simulink model "JMAP_Postfilt_SEModelv1d1"  (R2019a)
settings: Solver=FixedStepDiscrete  StartTime=0.0  StopTime=stopTime  RelTol=1e-3
InitFcn:
  | JMAP_INIT
StopFcn:
  | % Calls predefined matlab function for data analysis
  | JMAP_STOP
values from neighbouring files (symbols this model uses):
  aa = 0.98.*ones(FFT_size, 1)    [JMAP_INIT.m]    (also in JMAP_Postfilt_SE_OG.m = 0.98; JMAP_Postfilt_SE_v3.m = 0.98; JMAP_dataExport.m = 0.98; block_verScript.m = 0.98*ones(nSamp, FFT_size))
  beta = 2    [JMAP_INIT.m]    (also in JMAP_Postfilt_SE_OG.m; JMAP_dataExport.m; block_verScript.m = 2*ones(nSamp, FFT_size); ksi_verScript.m = 2*ones(nSamp, FFT_size))
  DPRAM1_size = FFT_size*2    (= 128)    [JMAP_INIT.m]
  FFT_frame_shift = FFT_size/4    (= 16)    [JMAP_INIT.m]
  FFT_size = 64    [FIR_filterTestm.m]    (also in JMAP_INIT.m; blockVerification.m; block_verScript.m; ksi_verScript.m)
  frameMag_initCond = abs(fft(sp(1:FFT_size), FFT_size))'    [JMAP_INIT.m]
  Fs = 48000    [FIR_filterTestm.m]    (also in JMAP_INIT.m; blockVerification.m; block_verScript.m; ksi_verScript.m)
  ksiInit = aa + (1-aa).*max(pSNR - 1, 0)    [JMAP_INIT.m]
  noiseVarianceInit = JMAP_noiseCalc(x)    [JMAP_INIT.m]
  SysRate_Upsample_Factor = 32    [JMAP_INIT.m]
  Ts = 1/Fs    (= 2.08333333333e-05)    [FIR_filterTestm.m]    (also in JMAP_INIT.m; blockVerification.m; block_verScript.m; ksi_verScript.m)
undefined symbols (not defined in the file or in its folder): Fs_in, magnitude
libraries: hdlsllib x16, simulink x7, dspxfrm3 x2, dspsigops x2
settings Model: Creator=Ross_admin  LastModifiedBy=Showi
settings DataIOCC: ReturnWorkspaceOutputs=off
settings OptimizationCC: BlockReduction=off  ConditionallyExecuteInputs=off  DefaultParameterBehavior=Inlined
settings DebuggingCC: AlgebraicLoopMsg=error  SingleTaskRateTransMsg=error  UnderSpecifiedDimensionMsg=warning  ArithmeticOperatorsInVariantConditions=warning
settings HardwareCC: ProdBitPerPointer=32  ProdBitPerSizeT=32  ProdBitPerPtrDiffT=32  ProdLargestAtomicFloat=None  ProdIntDivRoundTo=Undefined  ProdEndianess=Unspecified  ProdWordSize=32  ProdHWDeviceType=ASIC/FPGA->ASIC/FPGA  TargetBitPerPointer=64  TargetBitPerSizeT=64  TargetBitPerPtrDiffT=64  TargetLongLongMode=on  TargetIntDivRoundTo=Zero  TargetEndianess=LittleEndian  TargetWordSize=64  TargetHWDeviceType=Custom Processor->MATLAB Host Computer  ProdEqTarget=off
settings SFSimCC: SimUseLocalCustomCode=off
settings RTWCC: RTWUseLocalCustomCode=off
settings CodeAppCC: StateflowObjectComments=on

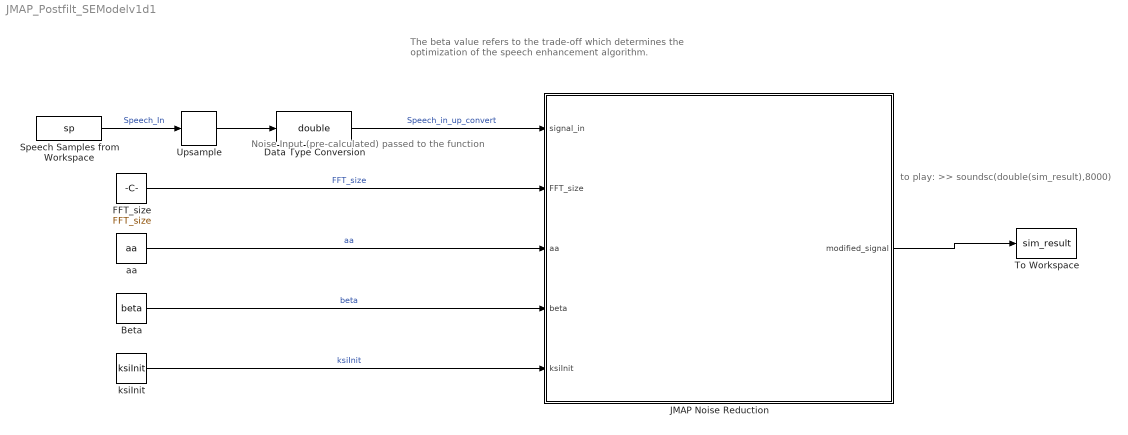
== system JMAP_Postfilt_SEModelv1d1 ==
  note: Noise Input (pre-calculated) passed to the function
  note: The beta value refers to the trade-off which determines the
      | optimization of the speech enhancement algorithm.
  note: to play: >> soundsc(double(sim_result),8000)
  Beta : Constant  Value=beta  SampleTime=Ts*2
  Data Type Conversion : DataTypeConversion  OutDataTypeStr=double
  FFT_size : Constant  Value=FFT_size  SampleTime=Ts*2
  JMAP Noise Reduction : Subsystem  TreatAsAtomicUnit=on
  Speech Samples from Workspace : FromWorkspace  VariableName=sp  SampleTime=Ts
  To Workspace : ToWorkspace  VariableName=sim_result  SampleTime=-1
  Upsample : dspsigops/Upsample  N=Fs/Fs_in  phase=0  RateOptions=Allow multirate processing  ic=0  mode=Unused parameter value
  aa : Constant  Value=aa  SampleTime=Ts*2
  ksiInit : Constant  Value=ksiInit  SampleTime=Ts*2
  wires:
  Speech Samples from Workspace/1 -> Upsample/1  "Speech_In"
  JMAP Noise Reduction/1(modified_signal) -> To Workspace/1
  Data Type Conversion/1 -> JMAP Noise Reduction/1(signal_in)  "Speech_in_up_convert"
  Upsample/1 -> Data Type Conversion/1
  Beta/1 -> JMAP Noise Reduction/4(beta)  "beta"
  aa/1 -> JMAP Noise Reduction/3(aa)  "aa"
  FFT_size/1 -> JMAP Noise Reduction/2(FFT_size)  "FFT_size"
  ksiInit/1 -> JMAP Noise Reduction/5(ksiInit)  "ksiInit"

== system JMAP_Postfilt_SEModelv1d1/JMAP Noise Reduction ==
  signal_in : Inport
  FFT_size : Inport  Port=2
  aa : Inport  Port=3
  beta : Inport  Port=4
  ksiInit : Inport  Port=5
  Analysis : Subsystem
  Frequency_Domain_Processing : Subsystem
  Synthesis : Subsystem
  modified_signal : Outport
  wires:
  signal_in/1 -> Analysis/1(Signal_in)
  Analysis/1(FFT_data) -> Frequency_Domain_Processing/5(FFT_results)
  Analysis/2(FFT_valid) -> Frequency_Domain_Processing/6(valid_in)
  Frequency_Domain_Processing/1(frequency_mods) -> Synthesis/1(FFT_data_mods)
  Frequency_Domain_Processing/2(valid_out) -> Synthesis/2(FFT_valid)
  Synthesis/1(modified_signal_out) -> modified_signal/1
  Analysis/3(FFT_frame_pulse) -> Synthesis/3(FFT_frame_pulse)  "FFT_framePulse"
  FFT_size/1 -> Frequency_Domain_Processing/1(FFT_size)
  aa/1 -> Frequency_Domain_Processing/2(aa)
  beta/1 -> Frequency_Domain_Processing/3(beta)
  ksiInit/1 -> Frequency_Domain_Processing/4(ksiInit)

== system JMAP_Postfilt_SEModelv1d1/JMAP Noise Reduction/Analysis ==
  note: Hanning window is applied
  Signal_in : Inport
  Data Type Conversion : DataTypeConversion  OutDataTypeStr=double
  FFT : dspxfrm3/FFT HDL Optimized  FFTLength=FFT_size  Architecture=Burst Radix 2  ComplexMultiplication=Use 4 multipliers and 2 adders  BitReversedOutput=off  BitReversedInput=off  Normalize=off  SimulateUsing=Code generation  RoundingMethod=Floor  ResetInputPort=off  StartOutputPort=off  EndOutputPort=off
      settings: SourceProductName=DSP System Toolbox  SourceProductBaseCode=DS
  FFT Frame Buffering : Subsystem
  Terminator6 : Terminator
  FFT_data : Outport
  FFT_valid : Outport  Port=2
  FFT_frame_pulse : Outport  Port=3
  wires:
  FFT/3 -> Terminator6/1
  FFT Frame Buffering/3(FFT_Frame_Start_Pulse) -> FFT_frame_pulse/1
  Signal_in/1 -> FFT Frame Buffering/1(Sample_Data_in)
  FFT Frame Buffering/2(Valid_to_FFT) -> FFT/2
  FFT Frame Buffering/1(Data_to_FFT) -> FFT/1
  Data Type Conversion/1 -> FFT_data/1
  FFT/2 -> FFT_valid/1
  FFT/1 -> Data Type Conversion/1

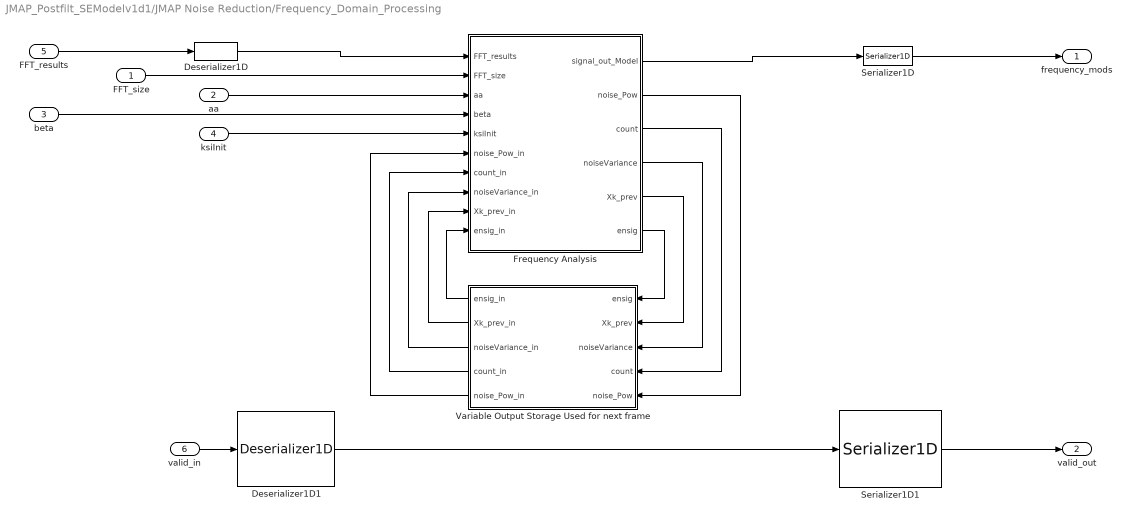
== system JMAP_Postfilt_SEModelv1d1/JMAP Noise Reduction/Frequency_Domain_Processing ==
  FFT_size : Inport
  aa : Inport  Port=2
  beta : Inport  Port=3
  ksiInit : Inport  Port=4
  FFT_results : Inport  Port=5
  valid_in : Inport  Port=6
  Deserializer1D : hdlsllib/HDL Operations/Deserializer1D  Ratio=FFT_size  IdleCycles=0  InitialCondition=0  startIn=off  validIn=off  validOut=off  inputDataDimensions=-1  inputSampleTime=-1  inputSignalType=auto
      settings: SourceProductName=HDL Coder  SourceProductBaseCode=HD
  Deserializer1D1 : hdlsllib/HDL Operations/Deserializer1D  Ratio=FFT_size  IdleCycles=0  InitialCondition=0  startIn=off  validIn=off  validOut=off  inputDataDimensions=-1  inputSampleTime=-1  inputSignalType=auto
      settings: SourceProductName=HDL Coder  SourceProductBaseCode=HD
  Frequency Analysis : Subsystem  TreatAsAtomicUnit=on
  Serializer1D : hdlsllib/HDL Operations/Serializer1D  Ratio=FFT_size  IdleCycles=0  validIn=off  startOut=off  validOut=off  inputDataDimensions=-1  inputSampleTime=-1  inputSignalType=auto
      settings: SourceProductName=HDL Coder  SourceProductBaseCode=HD
  Serializer1D1 : hdlsllib/HDL Operations/Serializer1D  Ratio=FFT_size  IdleCycles=0  validIn=off  startOut=off  validOut=off  inputDataDimensions=-1  inputSampleTime=-1  inputSignalType=auto
      settings: SourceProductName=HDL Coder  SourceProductBaseCode=HD
  Variable Output Storage Used for next frame : Subsystem
  frequency_mods : Outport
  valid_out : Outport  Port=2
  wires:
  Deserializer1D1/1 -> Serializer1D1/1
  FFT_results/1 -> Deserializer1D/1
  Serializer1D/1 -> frequency_mods/1
  valid_in/1 -> Deserializer1D1/1
  Serializer1D1/1 -> valid_out/1
  Deserializer1D/1 -> Frequency Analysis/1(FFT_results)
  Frequency Analysis/1(signal_out_Model) -> Serializer1D/1
  Frequency Analysis/6(ensig) -> Variable Output Storage Used for next frame/1(ensig)
  Frequency Analysis/5(Xk_prev) -> Variable Output Storage Used for next frame/2(Xk_prev)
  Frequency Analysis/4(noiseVariance) -> Variable Output Storage Used for next frame/3(noiseVariance)
  Frequency Analysis/3(count) -> Variable Output Storage Used for next frame/4(count)
  Variable Output Storage Used for next frame/1(ensig_in) -> Frequency Analysis/10(ensig_in)
  Variable Output Storage Used for next frame/2(Xk_prev_in) -> Frequency Analysis/9(Xk_prev_in)
  Variable Output Storage Used for next frame/3(noiseVariance_in) -> Frequency Analysis/8(noiseVariance_in)
  Variable Output Storage Used for next frame/4(count_in) -> Frequency Analysis/7(count_in)
  Frequency Analysis/2(noise_Pow) -> Variable Output Storage Used for next frame/5(noise_Pow)
  Variable Output Storage Used for next frame/5(noise_Pow_in) -> Frequency Analysis/6(noise_Pow_in)
  FFT_size/1 -> Frequency Analysis/2(FFT_size)
  beta/1 -> Frequency Analysis/4(beta)
  aa/1 -> Frequency Analysis/3(aa)
  ksiInit/1 -> Frequency Analysis/5(ksiInit)

== system JMAP_Postfilt_SEModelv1d1/JMAP Noise Reduction/Synthesis ==
  note: Making the assumption here
      | that the frequency domain processing
      | preserved the complex conjugate pairs.
  note: See Note 1
  note: Note 1:
      | Reshape is to avoid a simulink error.
      | Adding a FIFO to the iFFT block causes the
      | iFFT to change its output datatypes,
      | i.e. the data and valid signals
      | become a [1x1] matrix (Simulink Bug).
      | This work around was given by Mathworks
      | tech support (March 16, 2018).
      | Matlab 2017b
  note: See Note 1
  FFT_data_mods : Inport
  FFT_valid : Inport  Port=2
  FFT_frame_pulse : Inport  Port=3
  Data Type Conversion1 : DataTypeConversion  Commented=through  OutDataTypeStr=fixdt(1,Wbits,Fbits)
  Get_Real : ComplexToRealImag
  Overlap_and_Add : Subsystem
  Reshape : Reshape
  Reshape1 : Reshape
  Terminator8 : Terminator
  Terminator9 : Terminator
  iFFT : dspxfrm3/IFFT HDL Optimized  FFTLength=FFT_size  Architecture=Burst Radix 2  ComplexMultiplication=Use 4 multipliers and 2 adders  BitReversedOutput=off  BitReversedInput=off  Normalize=on  SimulateUsing=Code generation  RoundingMethod=Floor  ResetInputPort=off  StartOutputPort=off  EndOutputPort=off
      settings: SourceProductName=DSP System Toolbox  SourceProductBaseCode=DS
  modified_signal_out : Outport
  wires:
  iFFT/3 -> Terminator8/1
  Reshape1/1 -> Overlap_and_Add/2(iFFT_Valid)
  Reshape/1 -> Overlap_and_Add/1(IFFT_Data)
  iFFT/2 -> Reshape1/1
  Overlap_and_Add/1(signal_out) -> Data Type Conversion1/1
  FFT_data_mods/1 -> iFFT/1
  Data Type Conversion1/1 -> modified_signal_out/1  "modified_signal_outt"
  iFFT/1 -> Get_Real/1
  Get_Real/1 -> Reshape/1
  Get_Real/2 -> Terminator9/1
  FFT_valid/1 -> iFFT/2
  FFT_frame_pulse/1 -> Overlap_and_Add/3(FFT_Frame_Pulse)

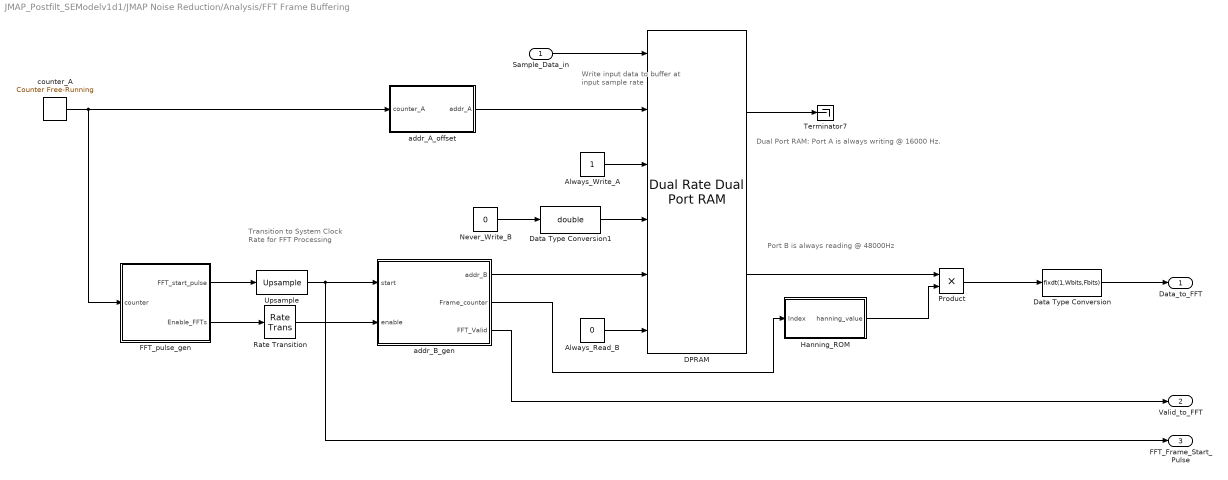
== system JMAP_Postfilt_SEModelv1d1/JMAP Noise Reduction/Analysis/FFT Frame Buffering ==
  note: Port B is always reading @ 48000Hz
  note: Dual Port RAM: Port A is always writing @ 16000 Hz.
  note: Transition to
      | System Clock Rate
      | for FFT Processing
  note: Write input data
      | to buffer at input
      | sample rate
  Sample_Data_in : Inport
  Always_Read_B : Constant  Value=0  OutDataTypeStr=boolean  SampleTime=Ts/SysRate_Upsample_Factor
  Always_Write_A : Constant  OutDataTypeStr=boolean  SampleTime=Ts
  DPRAM : hdlsllib/HDL RAMs/Dual Rate Dual Port RAM  ram_size=DPRAM1_address_size
      settings: SourceProductName=HDL Coder  SourceProductBaseCode=HD
  Data Type Conversion : DataTypeConversion  OutDataTypeStr=fixdt(1,Wbits,Fbits)
  Data Type Conversion1 : DataTypeConversion  OutDataTypeStr=double
  FFT_pulse_gen : Subsystem
  Hanning_ROM : Subsystem
  Never_Write_B : Constant  Value=0  OutDataTypeStr=fixdt(1,Wbits,Fbits)  SampleTime=Ts/SysRate_Upsample_Factor
  Product : Product
  Rate Transition : RateTransition  OutPortSampleTimeOpt=Multiple of input port sample time  OutPortSampleTimeMultiple=1/SysRate_Upsample_Factor
  Terminator7 : Terminator
  Upsample : dspsigops/Upsample  N=SysRate_Upsample_Factor  phase=0  RateOptions=Allow multirate processing  ic=0  mode=Unused parameter value
  addr_A_offset : Subsystem
  addr_B_gen : Subsystem
  counter_A : simulink/Sources/Counter Free-Running  NumBits=DPRAM1_address_size  tsamp=Ts
  Data_to_FFT : Outport
  Valid_to_FFT : Outport  Port=2
  FFT_Frame_Start_Pulse : Outport  Port=3
  wires:
  Always_Write_A/1 -> DPRAM/3
  Always_Read_B/1 -> DPRAM/6
  DPRAM/1 -> Terminator7/1
  addr_B_gen/3(FFT_Valid) -> Valid_to_FFT/1
  addr_B_gen/1(addr_B) -> DPRAM/5
  counter_A/1 -> addr_A_offset/1(counter_A), FFT_pulse_gen/1(counter)
  Sample_Data_in/1 -> DPRAM/1
  addr_A_offset/1(addr_A) -> DPRAM/2
  addr_B_gen/2(Frame_counter) -> Hanning_ROM/1(Index)
  Product/1 -> Data Type Conversion/1
  DPRAM/2 -> Product/1
  Hanning_ROM/1(hanning_value) -> Product/2
  Data Type Conversion/1 -> Data_to_FFT/1
  Rate Transition/1 -> addr_B_gen/2(enable)
  FFT_pulse_gen/1(FFT_start_pulse) -> Upsample/1
  FFT_pulse_gen/2(Enable_FFTs) -> Rate Transition/1
  Upsample/1 -> FFT_Frame_Start_Pulse/1, addr_B_gen/1(start)
  Data Type Conversion1/1 -> DPRAM/4
  Never_Write_B/1 -> Data Type Conversion1/1

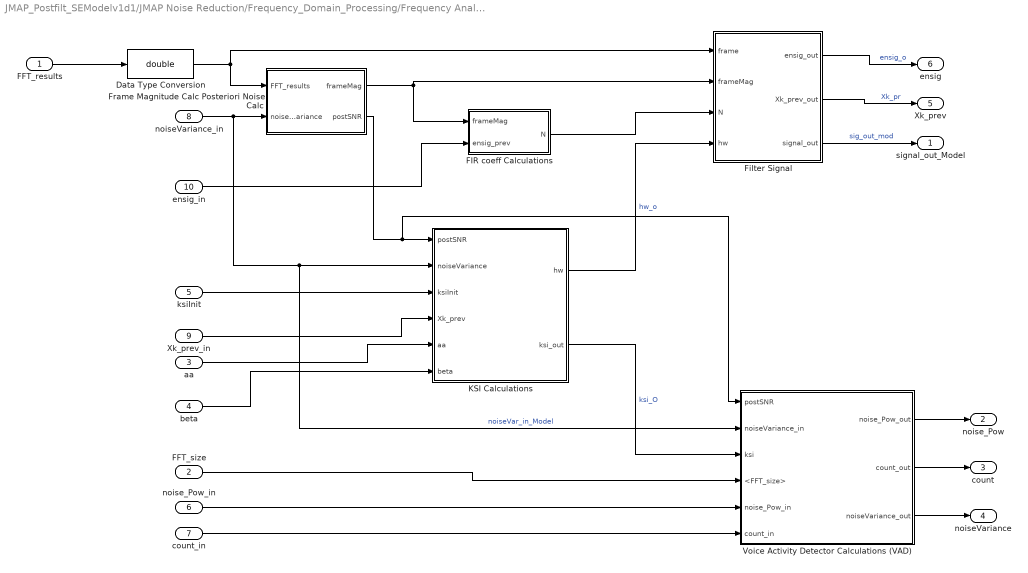
== system JMAP_Postfilt_SEModelv1d1/JMAP Noise Reduction/Frequency_Domain_Processing/Frequency Analysis ==
  FFT_results : Inport
  FFT_size : Inport  Port=2
  aa : Inport  Port=3
  beta : Inport  Port=4
  ksiInit : Inport  Port=5
  noise_Pow_in : Inport  Port=6
  count_in : Inport  Port=7
  noiseVariance_in : Inport  Port=8
  Xk_prev_in : Inport  Port=9
  ensig_in : Inport  Port=10
  Data Type Conversion : DataTypeConversion  OutDataTypeStr=double
  FIR coeff Calculations : Subsystem
  Filter Signal : Subsystem
  Frame Magnitude Calc Posteriori Noise Calc : Subsystem
  KSI Calculations : Subsystem
  Voice Activity Detector Calculations (VAD) : Subsystem
  signal_out_Model : Outport  InitialOutput=0
  noise_Pow : Outport  Port=2  InitialOutput=0
  count : Outport  Port=3  InitialOutput=0
  noiseVariance : Outport  Port=4  InitialOutput=0
  Xk_prev : Outport  Port=5  InitialOutput=0
  ensig : Outport  Port=6  InitialOutput=0
  wires:
  noise_Pow_in/1 -> Voice Activity Detector Calculations (VAD)/5("noise_Pow_in ")
  count_in/1 -> Voice Activity Detector Calculations (VAD)/6(count_in)
  Voice Activity Detector Calculations (VAD)/3(noiseVariance_out) -> noiseVariance/1
  Voice Activity Detector Calculations (VAD)/2(count_out) -> count/1
  Voice Activity Detector Calculations (VAD)/1(noise_Pow_out) -> noise_Pow/1
  Filter Signal/2(Xk_prev_out) -> Xk_prev/1  "Xk_pr"
  Filter Signal/1(ensig_out) -> ensig/1  "ensig_o"
  Filter Signal/3(signal_out) -> signal_out_Model/1  "sig_out_mod"
  Frame Magnitude Calc Posteriori Noise Calc/1(frameMag) -> FIR coeff Calculations/1(frameMag), Filter Signal/2(frameMag)
  FIR coeff Calculations/1(N) -> Filter Signal/3(N)
  Frame Magnitude Calc Posteriori Noise Calc/2(postSNR) -> Voice Activity Detector Calculations (VAD)/1(postSNR), KSI Calculations/1(postSNR)
  FFT_size/1 -> Voice Activity Detector Calculations (VAD)/4(<FFT_size>)
  Xk_prev_in/1 -> KSI Calculations/4(Xk_prev)
  aa/1 -> KSI Calculations/5(aa)
  beta/1 -> KSI Calculations/6(beta)
  KSI Calculations/1(hw) -> Filter Signal/4(hw)  "hw_o"
  KSI Calculations/2(ksi_out) -> Voice Activity Detector Calculations (VAD)/3(ksi)  "ksi_O"
  noiseVariance_in/1 -> KSI Calculations/2(noiseVariance), Voice Activity Detector Calculations (VAD)/2(noiseVariance_in), Frame Magnitude Calc Posteriori Noise Calc/2(noiseVariance)  "noiseVar_in_Model"
  FFT_results/1 -> Data Type Conversion/1
  Data Type Conversion/1 -> Filter Signal/1(frame), Frame Magnitude Calc Posteriori Noise Calc/1(FFT_results)
  ksiInit/1 -> KSI Calculations/3(ksiInit)
  ensig_in/1 -> FIR coeff Calculations/2(ensig_prev)

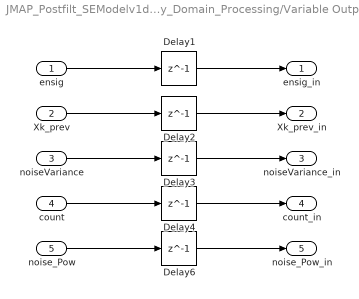
== system JMAP_Postfilt_SEModelv1d1/JMAP Noise Reduction/Frequency_Domain_Processing/Variable Output Storage Used for next frame ==
  ensig : Inport
  Xk_prev : Inport  Port=2
  noiseVariance : Inport  Port=3
  count : Inport  Port=4
  noise_Pow : Inport  Port=5
  Delay1 : Delay  DelayLength=1  InitialCondition=frameMag_initCond
  Delay2 : Delay  DelayLength=1  InitialCondition=zeros(FFT_size, 1)
  Delay3 : Delay  DelayLength=1  InitialCondition=noiseVarianceInit
  Delay4 : Delay  DelayLength=1  InitialCondition=1
  Delay6 : Delay  DelayLength=1  InitialCondition=zeros(FFT_size, 1)
  ensig_in : Outport
  Xk_prev_in : Outport  Port=2
  noiseVariance_in : Outport  Port=3
  count_in : Outport  Port=4
  noise_Pow_in : Outport  Port=5
  wires:
  ensig/1 -> Delay1/1
  Delay1/1 -> ensig_in/1
  Xk_prev/1 -> Delay2/1
  Delay2/1 -> Xk_prev_in/1
  noiseVariance/1 -> Delay3/1
  Delay3/1 -> noiseVariance_in/1
  count/1 -> Delay4/1
  Delay4/1 -> count_in/1
  noise_Pow/1 -> Delay6/1
  Delay6/1 -> noise_Pow_in/1

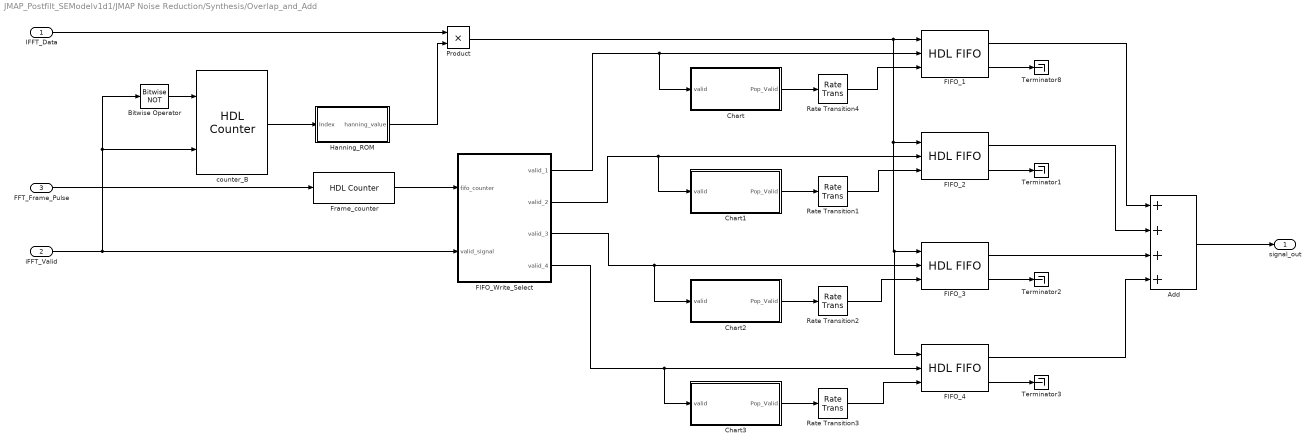
== system JMAP_Postfilt_SEModelv1d1/JMAP Noise Reduction/Synthesis/Overlap_and_Add ==
  IFFT_Data : Inport
  iFFT_Valid : Inport  Port=2
  FFT_Frame_Pulse : Inport  Port=3
  Add : Sum  Inputs=4
  Bitwise Operator : simulink/Logic and Bit Operations/Bitwise Operator  logicop=NOT  UseBitMask=off  BitMask=bin2dec('11011001')  BitMaskRealWorld=Stored Integer
  Chart : Stateflow chart  TreatAsAtomicUnit=on
  Chart1 : Stateflow chart  TreatAsAtomicUnit=on
  Chart2 : Stateflow chart  TreatAsAtomicUnit=on
  Chart3 : Stateflow chart  TreatAsAtomicUnit=on
  FIFO_{1..4} (4 alike) : hdlsllib/HDL RAMs/HDL FIFO  fifo_size=FFT_size  ratio=SysRate_Upsample_Factor  push_msg=Warning  pop_msg=Warning  show_empty=off  show_full=on  show_num=off
      settings: SourceProductName=HDL Coder  SourceProductBaseCode=HD
  FIFO_Write_Select : MATLAB Function  TreatAsAtomicUnit=on
  Frame_counter : hdlsllib/Sources/HDL Counter  CountType=Free running  CountInit=2  CountStep=1  CountMax=1024  CountFromType=Initial value  CountFrom=2  CountResetPort=off  CountLoadPort=off  CountEnbPort=on  CountDirPort=off  CountDataType=Unsigned  CountWordLen=2  CountFracLen=0  CountSampTime=1
      settings: SourceProductBaseCode=HD
  Hanning_ROM : Subsystem
  Product : Product
  Rate Transition{1..4} (4 alike) : RateTransition  OutPortSampleTimeOpt=Multiple of input port sample time  OutPortSampleTimeMultiple=SysRate_Upsample_Factor
  Terminator{1..3,8} (4 alike) : Terminator
  counter_B : hdlsllib/Sources/HDL Counter  CountType=Count limited  CountInit=0  CountStep=1  CountMax=FFT_size  CountFromType=Initial value  CountFrom=0  CountResetPort=on  CountLoadPort=off  CountEnbPort=on  CountDirPort=off  CountDataType=Unsigned  CountWordLen=DPRAM1_address_size  CountFracLen=0  CountSampTime=1
      settings: SourceProductBaseCode=HD
  signal_out : Outport
  wires:
  FIFO_1/1 -> Add/1
  FIFO_3/1 -> Add/3
  FFT_Frame_Pulse/1 -> Frame_counter/1
  FIFO_2/1 -> Add/2
  FIFO_Write_Select/3(valid_3) -> Chart2/1(valid), FIFO_3/2
  FIFO_Write_Select/4(valid_4) -> Chart3/1(valid), FIFO_4/2
  FIFO_4/1 -> Add/4
  FIFO_Write_Select/1(valid_1) -> FIFO_1/2, Chart/1(valid)
  FIFO_Write_Select/2(valid_2) -> FIFO_2/2, Chart1/1(valid)
  Add/1 -> signal_out/1
  Frame_counter/1 -> FIFO_Write_Select/1(fifo_counter)
  FIFO_4/2 -> Terminator3/1
  FIFO_2/2 -> Terminator1/1
  FIFO_3/2 -> Terminator2/1
  Bitwise Operator/1 -> counter_B/1
  iFFT_Valid/1 -> counter_B/2, Bitwise Operator/1, FIFO_Write_Select/2(valid_signal)
  IFFT_Data/1 -> Product/1
  Product/1 -> FIFO_4/1, FIFO_3/1, FIFO_2/1, FIFO_1/1
  Hanning_ROM/1(hanning_value) -> Product/2
  counter_B/1 -> Hanning_ROM/1(Index)
  Chart/1(Pop_Valid) -> Rate Transition4/1
  Rate Transition4/1 -> FIFO_1/3
  FIFO_1/2 -> Terminator8/1
  Chart1/1(Pop_Valid) -> Rate Transition1/1
  Rate Transition1/1 -> FIFO_2/3
  Chart2/1(Pop_Valid) -> Rate Transition2/1
  Rate Transition2/1 -> FIFO_3/3
  Chart3/1(Pop_Valid) -> Rate Transition3/1
  Rate Transition3/1 -> FIFO_4/3

== system JMAP_Postfilt_SEModelv1d1/JMAP Noise Reduction/Analysis/FFT Frame Buffering/FFT_pulse_gen ==
  note: Don't send out start pulses until
      | circular buffer has filled.
  counter : Inport
  FFT_Frame_Pulse_Gen : Subsystem
  Subsystem : Subsystem
  FFT_start_pulse : Outport
  Enable_FFTs : Outport  Port=2
  wires:
  counter/1 -> FFT_Frame_Pulse_Gen/1("counter_value ")
  Subsystem/1(FFT_Frame_Start) -> FFT_start_pulse/1
  Subsystem/2(Enable_FFT_Frames) -> Enable_FFTs/1
  FFT_Frame_Pulse_Gen/1(Frame_Pulse) -> Subsystem/1(Frame_Pulse)

== system JMAP_Postfilt_SEModelv1d1/JMAP Noise Reduction/Analysis/FFT Frame Buffering/Hanning_ROM ==
  Index : Inport
  Lookup Table : Lookup_n-D  NumberOfTableDimensions=1  BreakpointsForDimension1=[0:FFT_size]  IndexSearchMethod=Evenly spaced points  Table=hanning(FFT_size+1)  InterpMethod=Flat  ExtrapMethod=Clip  DiagnosticForOutOfRangeInput=Error  UseLastTableValue=on  OutDataTypeStr=double  RndMeth=Simplest  InputSameDT=on
  Unit Delay : UnitDelay  SampleTime=-1  HasFrameUpgradeWarning=on
  hanning_value : Outport
  wires:
  Unit Delay/1 -> hanning_value/1
  Index/1 -> Lookup Table/1
  Lookup Table/1 -> Unit Delay/1

== system JMAP_Postfilt_SEModelv1d1/JMAP Noise Reduction/Analysis/FFT Frame Buffering/addr_A_offset ==
  note: Add 1 to counter since the read pointer (addr_B)
      | can catch the write pointer (addr_A) if
      | SysRate_Upsample_Factor is large enough
  counter_A : Inport
  Add : Sum  OutDataTypeStr=fixdt(0,DPRAM1_address_size,0)
  write_offset : Constant  OutDataTypeStr=fixdt(0,DPRAM1_address_size,0)  SampleTime=Ts
  addr_A : Outport
  wires:
  write_offset/1 -> Add/2
  Add/1 -> addr_A/1
  counter_A/1 -> Add/1

== system JMAP_Postfilt_SEModelv1d1/JMAP Noise Reduction/Analysis/FFT Frame Buffering/addr_B_gen ==
  start : Inport
  enable : Inport  Port=2
  Logical Operator1 : Logic  AllPortsSameDT=off  OutDataTypeStr=boolean
  addr_B_gen_enable : Subsystem
  counter_B : hdlsllib/Sources/HDL Counter  CountType=Free running  CountInit=DPRAM1_size-10  CountStep=1  CountMax=1024  CountFromType=Initial value  CountFrom=DPRAM1_size-10  CountResetPort=off  CountLoadPort=on  CountEnbPort=on  CountDirPort=off  CountDataType=Unsigned  CountWordLen=DPRAM1_address_size  CountFracLen=0  CountSampTime=1
      settings: SourceProductBaseCode=HD
  addr_B : Outport
  Frame_counter : Outport  Port=2
  FFT_Valid : Outport  Port=3
  wires:
  counter_B/1 -> addr_B/1
  start/1 -> counter_B/1, addr_B_gen_enable/1(start)
  addr_B_gen_enable/1(enable_B) -> Logical Operator1/1
  addr_B_gen_enable/2(Start_Address) -> counter_B/2
  enable/1 -> Logical Operator1/2
  addr_B_gen_enable/3(Frame_Index) -> Frame_counter/1
  Logical Operator1/1 -> FFT_Valid/1, counter_B/3

== system JMAP_Postfilt_SEModelv1d1/JMAP Noise Reduction/Frequency_Domain_Processing/Frequency Analysis/FIR coeff Calculations ==
  frameMag : Inport
  ensig_prev : Inport  Port=2
  Calculate Coeffs and Filter Length : Subsystem
  PR Calculations : Subsystem
  PRT Calculation : Subsystem
  N : Outport
  wires:
  ensig_prev/1 -> PR Calculations/1(ensig_prev)
  PR Calculations/1(PR) -> PRT Calculation/1(PR)
  Calculate Coeffs and Filter Length/1(N) -> N/1
  PRT Calculation/1(PRT) -> Calculate Coeffs and Filter Length/1(PRT)
  frameMag/1 -> PR Calculations/2(frameMag)

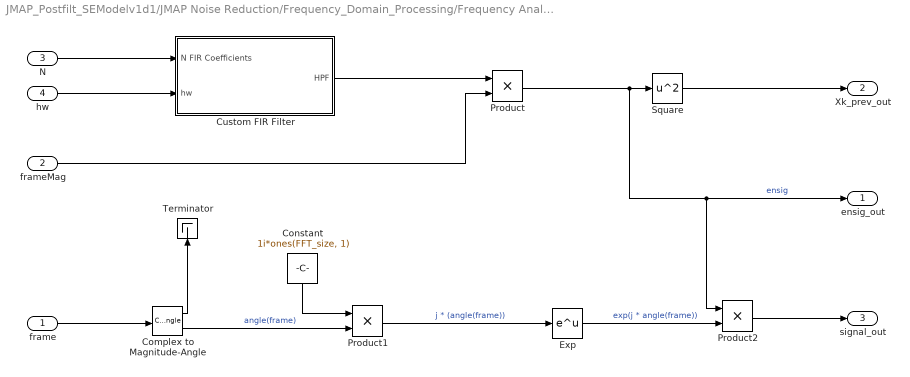
== system JMAP_Postfilt_SEModelv1d1/JMAP Noise Reduction/Frequency_Domain_Processing/Frequency Analysis/Filter Signal ==
  frame : Inport
  frameMag : Inport  Port=2
  N : Inport  Port=3
  hw : Inport  Port=4
  Complex to Magnitude-Angle : ComplexToMagnitudeAngle
  Constant : Constant  Value=1i*ones(FFT_size, 1)  SampleTime=-1
  Custom FIR Filter : Subsystem
  Exp : Math  SaturateOnIntegerOverflow=on
  Product : Product
  Product1 : Product
  Product2 : Product
  Square : Math  Operator=square  RndMeth=Zero  SaturateOnIntegerOverflow=on
  Terminator : Terminator
  ensig_out : Outport
  Xk_prev_out : Outport  Port=2
  signal_out : Outport  Port=3
  wires:
  Square/1 -> Xk_prev_out/1
  frameMag/1 -> Product/2
  Product1/1 -> Exp/1  "j * (angle(frame))"
  Constant/1 -> Product1/1
  Exp/1 -> Product2/2  "exp(j * angle(frame))"
  Product2/1 -> signal_out/1
  Complex to Magnitude-Angle/2 -> Product1/2  "angle(frame)"
  Complex to Magnitude-Angle/1 -> Terminator/1
  N/1 -> Custom FIR Filter/1(N FIR Coefficients)
  hw/1 -> Custom FIR Filter/2(hw)
  frame/1 -> Complex to Magnitude-Angle/1
  Product/1 -> Product2/1, ensig_out/1, Square/1  "ensig"
  Custom FIR Filter/1(HPF) -> Product/1

== system JMAP_Postfilt_SEModelv1d1/JMAP Noise Reduction/Frequency_Domain_Processing/Frequency Analysis/Frame Magnitude Calc Posteriori Noise Calc ==
  FFT_results : Inport
  noiseVariance : Inport  Port=2
  Subsystem1 : Subsystem
  Subsystem3 : Subsystem
  frameMag : Outport
  postSNR : Outport  Port=2
  wires:
  Subsystem3/2(frameMag) -> frameMag/1
  Subsystem3/1(framePower) -> Subsystem1/1(framePower)
  FFT_results/1 -> Subsystem3/1(FFT_results)
  noiseVariance/1 -> Subsystem1/2(noiseVariance)
  Subsystem1/1(postSNR) -> postSNR/1  "postSNR"

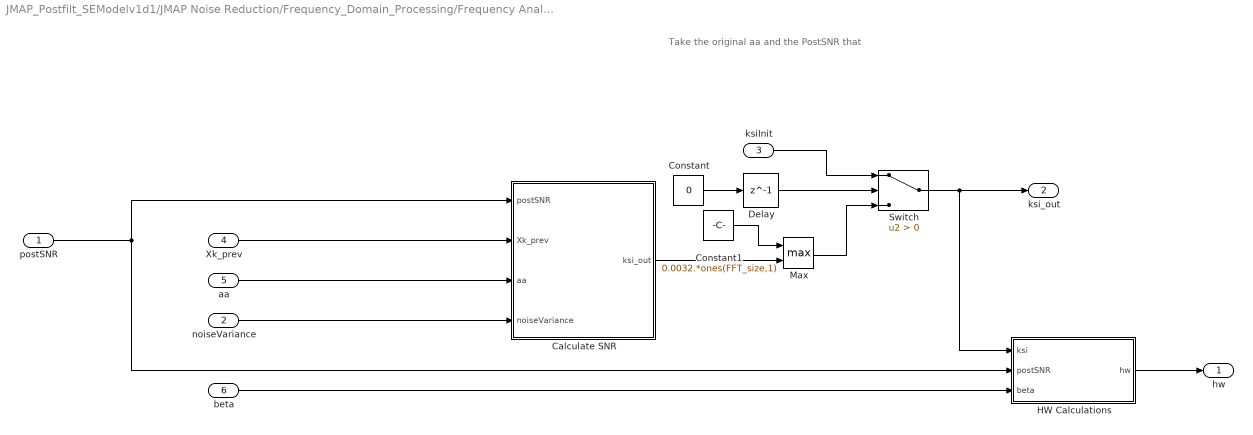
== system JMAP_Postfilt_SEModelv1d1/JMAP Noise Reduction/Frequency_Domain_Processing/Frequency Analysis/KSI Calculations ==
  note: Take the original aa and the PostSNR that
  postSNR : Inport
  noiseVariance : Inport  Port=2
  ksiInit : Inport  Port=3
  Xk_prev : Inport  Port=4
  aa : Inport  Port=5
  beta : Inport  Port=6
  Calculate SNR : Subsystem
  Constant : Constant  Value=0  SampleTime=-1
  Constant1 : Constant  Value=0.0032.*ones(FFT_size,1)  SampleTime=-1
  Delay : Delay  DelayLength=1  InitialCondition=1
  HW Calculations : Subsystem
  Max : MinMax  Function=max  Inputs=2
  Switch : Switch  Criteria=u2 > Threshold
  hw : Outport
  ksi_out : Outport  Port=2
  wires:
  noiseVariance/1 -> Calculate SNR/4(noiseVariance)
  beta/1 -> HW Calculations/3(beta)
  postSNR/1 -> HW Calculations/2(postSNR), Calculate SNR/1(postSNR)
  Xk_prev/1 -> Calculate SNR/2(Xk_prev)
  aa/1 -> Calculate SNR/3(aa)
  HW Calculations/1(hw) -> hw/1
  Switch/1 -> HW Calculations/1(ksi), ksi_out/1
  ksiInit/1 -> Switch/1
  Delay/1 -> Switch/2
  Constant/1 -> Delay/1
  Calculate SNR/1(ksi_out) -> Max/2
  Constant1/1 -> Max/1
  Max/1 -> Switch/3

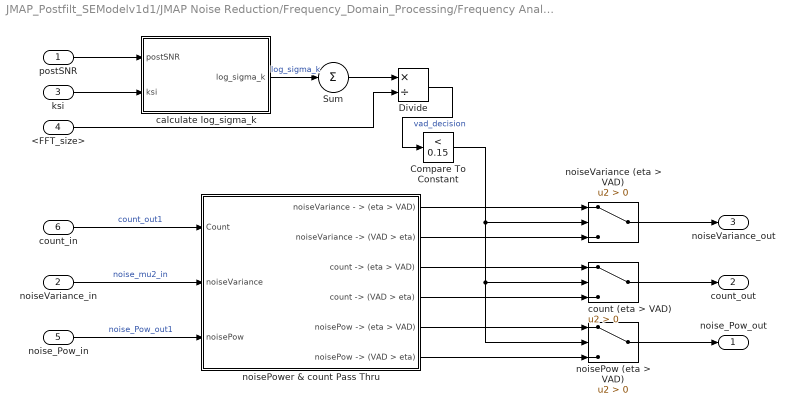
== system JMAP_Postfilt_SEModelv1d1/JMAP Noise Reduction/Frequency_Domain_Processing/Frequency Analysis/Voice Activity Detector Calculations (VAD) ==
  postSNR : Inport
  noiseVariance_in : Inport  Port=2
  ksi : Inport  Port=3
  <FFT_size> : Inport  Port=4
  "noise_Pow_in " : Inport  Port=5
  count_in : Inport  Port=6
  Compare To Constant : simulink/Logic and Bit Operations/Compare To Constant  relop=<  const=0.15  OutDataTypeStr=boolean
  Divide : Product  Inputs=*/  SaturateOnIntegerOverflow=on  RndMeth=Zero
  Sum : Sum  Inputs=+
  calculate log_sigma_k : Subsystem
  count (eta > VAD) : Switch  Criteria=u2 > Threshold
  noisePow (eta > VAD) : Switch  Criteria=u2 > Threshold
  noisePower & count Pass Thru : Subsystem
  noiseVariance (eta > VAD) : Switch  Criteria=u2 > Threshold
  noise_Pow_out : Outport  InitialOutput=0
  count_out : Outport  Port=2
  noiseVariance_out : Outport  Port=3
  wires:
  postSNR/1 -> calculate log_sigma_k/1(postSNR)
  ksi/1 -> calculate log_sigma_k/2(ksi)
  calculate log_sigma_k/1(log_sigma_k) -> Sum/1  "log_sigma_k"
  Sum/1 -> Divide/1
  <FFT_size>/1 -> Divide/2
  Divide/1 -> Compare To Constant/1  "vad_decision"
  noiseVariance_in/1 -> noisePower & count Pass Thru/2(noiseVariance)  "noise_mu2_in"
  "noise_Pow_in "/1 -> noisePower & count Pass Thru/3(noisePow)  "noise_Pow_out1"
  count_in/1 -> noisePower & count Pass Thru/1(Count)  "count_out1"
  Compare To Constant/1 -> noisePow (eta > VAD)/2, count (eta > VAD)/2, noiseVariance (eta > VAD)/2
  noisePower & count Pass Thru/1(noiseVariance - > (eta > VAD)) -> noiseVariance (eta > VAD)/1
  noisePower & count Pass Thru/2("noiseVariance -> (VAD > eta)") -> noiseVariance (eta > VAD)/3
  noisePower & count Pass Thru/3("count -> (eta > VAD)") -> count (eta > VAD)/1
  noisePower & count Pass Thru/4("count -> (VAD > eta)") -> count (eta > VAD)/3
  noiseVariance (eta > VAD)/1 -> noiseVariance_out/1
  count (eta > VAD)/1 -> count_out/1
  noisePow (eta > VAD)/1 -> noise_Pow_out/1
  noisePower & count Pass Thru/5("noisePow -> (eta > VAD)") -> noisePow (eta > VAD)/1
  noisePower & count Pass Thru/6("noisePow -> (VAD > eta)") -> noisePow (eta > VAD)/3

== system JMAP_Postfilt_SEModelv1d1/JMAP Noise Reduction/Synthesis/Overlap_and_Add/Hanning_ROM ==
  Index : Inport
  Lookup Table : Lookup_n-D  NumberOfTableDimensions=1  BreakpointsForDimension1=[0:FFT_size]  IndexSearchMethod=Evenly spaced points  Table=hanning(FFT_size+1)  InterpMethod=Flat  ExtrapMethod=Clip  DiagnosticForOutOfRangeInput=Error  UseLastTableValue=on  OutDataTypeStr=double  RndMeth=Simplest  InputSameDT=on
  Unit Delay : UnitDelay  SampleTime=-1  HasFrameUpgradeWarning=on
  hanning_value : Outport
  wires:
  Unit Delay/1 -> hanning_value/1
  Index/1 -> Lookup Table/1
  Lookup Table/1 -> Unit Delay/1

== system JMAP_Postfilt_SEModelv1d1/JMAP Noise Reduction/Analysis/FFT Frame Buffering/FFT_pulse_gen/FFT_Frame_Pulse_Gen ==
  "counter_value " : Inport
  Bit Slice : hdlsllib/Logic and Bit Operations/Bit Slice  lidx=log2(FFT_frame_shift)-1  ridx=0
  Compare To Zero : simulink/Logic and Bit Operations/Compare To Zero  relop===  OutDataTypeStr=boolean
  Frame_Pulse : Outport
  wires:
  "counter_value "/1 -> Bit Slice/1
  Compare To Zero/1 -> Frame_Pulse/1
  Bit Slice/1 -> Compare To Zero/1

== system JMAP_Postfilt_SEModelv1d1/JMAP Noise Reduction/Analysis/FFT Frame Buffering/FFT_pulse_gen/Subsystem ==
  note: Number of Frames
      | to wait before starting
  note: Start performing FFTs after enough data has filled the circular buffer.
      | This is due to the fact that we don't want the read pointer (addr_B)
      | to catch up with the  write pointer (addr_A) because if it does,
      | the DPRAM will throw an assertion error.
  Frame_Pulse : Inport
  Bitwise Operator : simulink/Logic and Bit Operations/Bitwise Operator  logicop=NOT  UseBitMask=off  BitMask=bin2dec('11011001')  BitMaskRealWorld=Stored Integer
  Compare To Constant : simulink/Logic and Bit Operations/Compare To Constant  relop=<  const=4  OutDataTypeStr=boolean
  Initial_frame_count : hdlsllib/Sources/HDL Counter  CountType=Count limited  CountInit=0  CountStep=1  CountMax=4  CountFromType=Specify  CountFrom=0  CountResetPort=off  CountLoadPort=off  CountEnbPort=on  CountDirPort=off  CountDataType=Unsigned  CountWordLen=5  CountFracLen=0  CountSampTime=1
      settings: SourceProductBaseCode=HD
  Logical Operator : Logic  AllPortsSameDT=off  OutDataTypeStr=boolean
  Logical Operator1 : Logic  AllPortsSameDT=off  OutDataTypeStr=boolean
  FFT_Frame_Start : Outport
  Enable_FFT_Frames : Outport  Port=2
  wires:
  Logical Operator1/1 -> FFT_Frame_Start/1
  Frame_Pulse/1 -> Logical Operator/2, Logical Operator1/1
  Initial_frame_count/1 -> Compare To Constant/1
  Logical Operator/1 -> Initial_frame_count/1
  Compare To Constant/1 -> Bitwise Operator/1, Logical Operator/1
  Bitwise Operator/1 -> Enable_FFT_Frames/1, Logical Operator1/2

== system JMAP_Postfilt_SEModelv1d1/JMAP Noise Reduction/Analysis/FFT Frame Buffering/addr_B_gen/addr_B_gen_enable ==
  start : Inport
  B_Enable_Counter : hdlsllib/Sources/HDL Counter  CountType=Count limited  CountInit=0  CountStep=1  CountMax=FFT_size  CountFromType=Specify  CountFrom=0  CountResetPort=on  CountLoadPort=off  CountEnbPort=on  CountDirPort=off  CountDataType=Unsigned  CountWordLen=DPRAM1_address_size  CountFracLen=0  CountSampTime=1
      settings: SourceProductBaseCode=HD
  Constant5 : Constant  Value=FFT_size  OutDataTypeStr=fixdt(0,11,0)  SampleTime=Ts/SysRate_Upsample_Factor
  Relational Operator : RelationalOperator  Operator=<  OutDataTypeStr=boolean  ZeroCross=off  RndMeth=Nearest
  Start_Address_Counter : hdlsllib/Sources/HDL Counter  CountType=Free running  CountInit=0  CountStep=FFT_frame_shift  CountMax=DPRAM1_size  CountFromType=Initial value  CountFrom=0  CountResetPort=off  CountLoadPort=off  CountEnbPort=on  CountDirPort=off  CountDataType=Unsigned  CountWordLen=DPRAM1_address_size  CountFracLen=0  CountSampTime=1
      settings: SourceProductBaseCode=HD
  enable_B : Outport
  Start_Address : Outport  Port=2
  Frame_Index : Outport  Port=3
  wires:
  Relational Operator/1 -> enable_B/1, B_Enable_Counter/2
  Constant5/1 -> Relational Operator/2
  B_Enable_Counter/1 -> Frame_Index/1, Relational Operator/1
  start/1 -> Start_Address_Counter/1, B_Enable_Counter/1
  Start_Address_Counter/1 -> Start_Address/1

== system JMAP_Postfilt_SEModelv1d1/JMAP Noise Reduction/Frequency_Domain_Processing/Frequency Analysis/FIR coeff Calculations/Calculate Coeffs and Filter Length ==
  PRT : Inport
  Compare To Constant : simulink/Logic and Bit Operations/Compare To Constant  relop===  const=1  OutDataTypeStr=boolean
  Constant : Constant  SampleTime=-1
  Enabled Subsystem1 : Subsystem  TreatAsAtomicUnit=on
  Switch : Switch  Criteria=u2 > Threshold
  N : Outport
  wires:
  PRT/1 -> Compare To Constant/1, Enabled Subsystem1/1(PRT)
  Compare To Constant/1 -> Switch/2
  Constant/1 -> Switch/1
  Enabled Subsystem1/1(N) -> Switch/3
  Switch/1 -> N/1

== system JMAP_Postfilt_SEModelv1d1/JMAP Noise Reduction/Frequency_Domain_Processing/Frequency Analysis/FIR coeff Calculations/PR Calculations ==
  ensig_prev : Inport
  frameMag : Inport  Port=2
  Add : Sum  Inputs=+
  Add1 : Sum  Inputs=+
  Add2 : Sum
  Constant : Constant  Value=eps  SampleTime=-1
  Divide : Product  Inputs=*/  SaturateOnIntegerOverflow=on  RndMeth=Zero
  Magnitude Squared : Math  Operator=magnitude^2  SaturateOnIntegerOverflow=on
  Magnitude Squared1 : Math  Operator=magnitude^2  SaturateOnIntegerOverflow=on
  PR : Outport
  wires:
  Magnitude Squared/1 -> Add/1
  ensig_prev/1 -> Magnitude Squared/1
  Add/1 -> Divide/1
  Magnitude Squared1/1 -> Add1/1
  frameMag/1 -> Magnitude Squared1/1
  Add1/1 -> Add2/1
  Constant/1 -> Add2/2
  Add2/1 -> Divide/2
  Divide/1 -> PR/1

== system JMAP_Postfilt_SEModelv1d1/JMAP Noise Reduction/Frequency_Domain_Processing/Frequency Analysis/FIR coeff Calculations/PRT Calculation ==
  PR : Inport
  Constant : Constant  SampleTime=-1
  Switch : Switch  Threshold=0.4
  PRT : Outport
  wires:
  PR/1 -> Switch/3, Switch/2
  Constant/1 -> Switch/1
  Switch/1 -> PRT/1

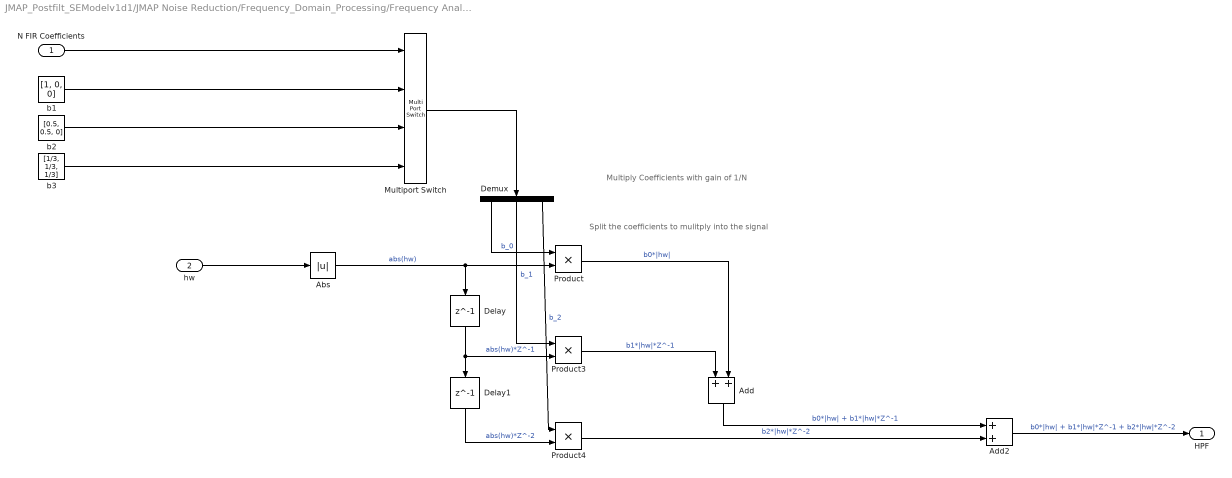
== system JMAP_Postfilt_SEModelv1d1/JMAP Noise Reduction/Frequency_Domain_Processing/Frequency Analysis/Filter Signal/Custom FIR Filter ==
  note: Split the coefficients to mulitply into the signal
  note: Multiply Coefficients with gain of 1/N
  N FIR Coefficients : Inport
  hw : Inport  Port=2
  Abs : Abs
  Add : Sum
  Add2 : Sum
  Delay : Delay  DelayLength=1
  Delay1 : Delay  DelayLength=1
  Demux : Demux  Outputs=3
  Multiport Switch : MultiPortSwitch  DiagnosticForDefault=Warning
  Product : Product
  Product3 : Product
  Product4 : Product
  b1 : Constant  Value=[1, 0, 0]  SampleTime=-1
  b2 : Constant  Value=[0.5, 0.5, 0]  SampleTime=-1
  b3 : Constant  Value=[1/3, 1/3, 1/3]  SampleTime=-1
  HPF : Outport
  wires:
  Delay/1 -> Delay1/1, Product3/2  "abs(hw)*Z^-1"
  Product/1 -> Add/2  "b0*|hw|"
  Product3/1 -> Add/1  "b1*|hw|*Z^-1"
  Abs/1 -> Product/2, Delay/1  "abs(hw)"
  Product4/1 -> Add2/2  "b2*|hw|*Z^-2"
  hw/1 -> Abs/1
  Delay1/1 -> Product4/2  "abs(hw)*Z^-2"
  Demux/3 -> Product4/1  "b_2"
  Demux/2 -> Product3/1  "b_1"
  Demux/1 -> Product/1  "b_0"
  Add/1 -> Add2/1  "b0*|hw| + b1*|hw|*Z^-1"
  Add2/1 -> HPF/1  "b0*|hw| + b1*|hw|*Z^-1 + b2*|hw|*Z^-2"
  N FIR Coefficients/1 -> Multiport Switch/1
  b1/1 -> Multiport Switch/2
  b2/1 -> Multiport Switch/3
  b3/1 -> Multiport Switch/4
  Multiport Switch/1 -> Demux/1

== system JMAP_Postfilt_SEModelv1d1/JMAP Noise Reduction/Frequency_Domain_Processing/Frequency Analysis/Frame Magnitude Calc Posteriori Noise Calc/Subsystem1 ==
  note: check max min value set from code
  framePower : Inport
  noiseVariance : Inport  Port=2
  Add : Sum
  Constant : Constant  Value=eps*ones(FFT_size, 1)  SampleTime=-1
  Constant1 : Constant  Value=40*ones(FFT_size, 1)  SampleTime=-1
  Divide : Product  Inputs=*/  SaturateOnIntegerOverflow=on  RndMeth=Zero
  Min : MinMax  Inputs=2
  postSNR : Outport
  wires:
  noiseVariance/1 -> Divide/2
  framePower/1 -> Divide/1
  Divide/1 -> Min/1  "postSNR"
  Constant1/1 -> Min/2
  Min/1 -> Add/1
  Add/1 -> postSNR/1
  Constant/1 -> Add/2

== system JMAP_Postfilt_SEModelv1d1/JMAP Noise Reduction/Frequency_Domain_Processing/Frequency Analysis/Frame Magnitude Calc Posteriori Noise Calc/Subsystem3 ==
  FFT_results : Inport
  Abs : Abs
  Square : Math  Operator=square  RndMeth=Zero  SaturateOnIntegerOverflow=on
  framePower : Outport
  frameMag : Outport  Port=2
  wires:
  Square/1 -> framePower/1  "framePower"
  Abs/1 -> frameMag/1, Square/1  "frameMag"
  FFT_results/1 -> Abs/1

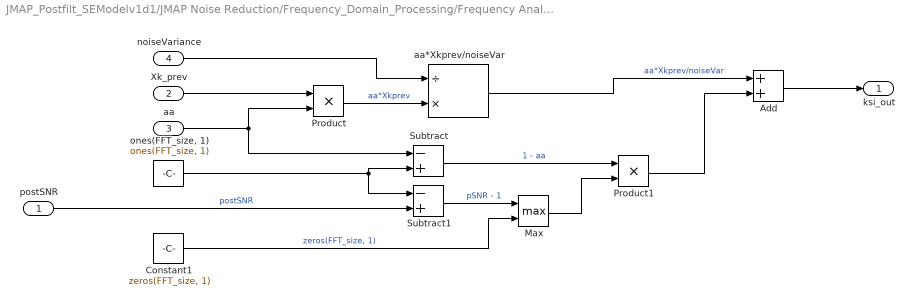
== system JMAP_Postfilt_SEModelv1d1/JMAP Noise Reduction/Frequency_Domain_Processing/Frequency Analysis/KSI Calculations/Calculate SNR ==
  postSNR : Inport
  Xk_prev : Inport  Port=2
  aa : Inport  Port=3
  noiseVariance : Inport  Port=4
  Add : Sum
  Constant1 : Constant  Value=zeros(FFT_size, 1)  SampleTime=-1
  Max : MinMax  Function=max  Inputs=2
  Product : Product
  Product1 : Product
  Subtract : Sum  Inputs=-+
  Subtract1 : Sum  Inputs=-+
  aa*Xkprev/noiseVar : Product  Inputs=/*  SaturateOnIntegerOverflow=on  RndMeth=Zero
  "ones(FFT_size, 1)" : Constant  Value=ones(FFT_size, 1)  SampleTime=-1
  ksi_out : Outport
  wires:
  Add/1 -> ksi_out/1
  Xk_prev/1 -> Product/1
  aa/1 -> Subtract/1, Product/2
  Product/1 -> aa*Xkprev/noiseVar/2  "aa*Xkprev"
  noiseVariance/1 -> aa*Xkprev/noiseVar/1
  "ones(FFT_size, 1)"/1 -> Subtract/2, Subtract1/1
  postSNR/1 -> Subtract1/2  "postSNR"
  Subtract/1 -> Product1/1  "1 - aa"
  Subtract1/1 -> Max/1  "pSNR - 1"
  Max/1 -> Product1/2
  Product1/1 -> Add/2
  aa*Xkprev/noiseVar/1 -> Add/1  "aa*Xkprev/noiseVar"
  Constant1/1 -> Max/2  "zeros(FFT_size, 1)"

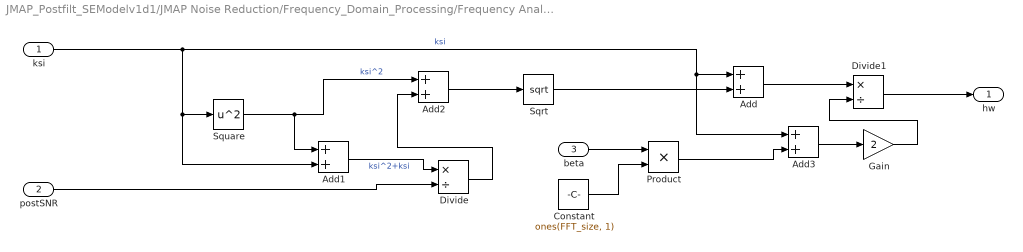
== system JMAP_Postfilt_SEModelv1d1/JMAP Noise Reduction/Frequency_Domain_Processing/Frequency Analysis/KSI Calculations/HW Calculations ==
  ksi : Inport
  postSNR : Inport  Port=2
  beta : Inport  Port=3
  Add{,1..3} (4 alike) : Sum
  Constant : Constant  Value=ones(FFT_size, 1)  SampleTime=Ts*2
  Divide : Product  Inputs=*/  SaturateOnIntegerOverflow=on  RndMeth=Zero
  Divide1 : Product  Inputs=*/  SaturateOnIntegerOverflow=on  RndMeth=Zero
  Gain : Gain  Gain=2
  Product : Product
  Sqrt : Sqrt  SaturateOnIntegerOverflow=on
  Square : Math  Operator=square  RndMeth=Zero  SaturateOnIntegerOverflow=on
  hw : Outport
  wires:
  ksi/1 -> Square/1, Add1/2, Add3/1, Add/1  "ksi"
  Square/1 -> Add2/1, Add1/1  "ksi^2"
  Sqrt/1 -> Add/2
  Add2/1 -> Sqrt/1
  beta/1 -> Product/1
  Add3/1 -> Gain/1
  Divide1/1 -> hw/1
  Add/1 -> Divide1/1
  Gain/1 -> Divide1/2
  postSNR/1 -> Divide/2
  Add1/1 -> Divide/1  "ksi^2+ksi"
  Divide/1 -> Add2/2
  Constant/1 -> Product/2
  Product/1 -> Add3/2

== system JMAP_Postfilt_SEModelv1d1/JMAP Noise Reduction/Frequency_Domain_Processing/Frequency Analysis/Voice Activity Detector Calculations (VAD)/calculate log_sigma_k ==
  postSNR : Inport
  ksi : Inport  Port=2
  Add : Sum
  Constant : Constant  Value=ones(FFT_size, 1)  SampleTime=-1
  Divide : Product  Inputs=*/  SaturateOnIntegerOverflow=on  RndMeth=Zero
  Product : Product
  Subtract : Sum  Inputs=+-
  ln : Math  Operator=log  SaturateOnIntegerOverflow=on
  log_sigma_k : Outport
  wires:
  ksi/1 -> Add/1, Product/2
  Constant/1 -> Add/2
  postSNR/1 -> Product/1
  Product/1 -> Divide/1
  Add/1 -> Divide/2, ln/1
  Divide/1 -> Subtract/1
  Subtract/1 -> log_sigma_k/1
  ln/1 -> Subtract/2

== system JMAP_Postfilt_SEModelv1d1/JMAP Noise Reduction/Frequency_Domain_Processing/Frequency Analysis/Voice Activity Detector Calculations (VAD)/noisePower & count Pass Thru ==
  Count : Inport
  noiseVariance : Inport  Port=2
  noisePow : Inport  Port=3
  Add : Sum
  Add1 : Sum
  Constant : Constant  SampleTime=-1
  Divide : Product  Inputs=/*  SaturateOnIntegerOverflow=on  RndMeth=Zero
  Divide1 : Product  Inputs=/*  SaturateOnIntegerOverflow=on  RndMeth=Zero
  noiseVariance - > (eta > VAD) : Outport
  "noiseVariance -> (VAD > eta)" : Outport  Port=2
  "count -> (eta > VAD)" : Outport  Port=3
  "count -> (VAD > eta)" : Outport  Port=4
  "noisePow -> (eta > VAD)" : Outport  Port=5
  "noisePow -> (VAD > eta)" : Outport  Port=6
  wires:
  noiseVariance/1 -> Add/1
  noisePow/1 -> Add/2, "noisePow -> (VAD > eta)"/1, Divide1/2  "VAD > eta"
  Count/1 -> Add1/2, "count -> (VAD > eta)"/1, Divide1/1  "count -> (VAD > eta)"
  Constant/1 -> Add1/1
  Add/1 -> "noisePow -> (eta > VAD)"/1, Divide/2  "noisePow -> (eta > VAD)"
  Add1/1 -> "count -> (eta > VAD)"/1, Divide/1  "count -> (eta > VAD)"
  Divide/1 -> noiseVariance - > (eta > VAD)/1  "nVar -> (eta > VAD)"
  Divide1/1 -> "noiseVariance -> (VAD > eta)"/1  "nVar -> (VAD > eta)"

== system JMAP_Postfilt_SEModelv1d1/JMAP Noise Reduction/Frequency_Domain_Processing/Frequency Analysis/FIR coeff Calculations/Calculate Coeffs and Filter Length/Enabled Subsystem1 ==
  PRT : Inport
  Constant : Constant  SampleTime=-1
  Constant1 : Constant  Value=0.4  SampleTime=-1
  Divide : Product  Inputs=*/  SaturateOnIntegerOverflow=on  RndMeth=Zero
  Gain : Gain  Gain=2
  Round : Rounding  Operator=round
  Subtract : Sum  Inputs=-+
  add : Sum
  N : Outport  InitialOutput=0
  wires:
  Gain/1 -> add/1
  PRT/1 -> Divide/1
  Constant/1 -> add/2, Subtract/2
  Subtract/1 -> Round/1
  Constant1/1 -> Divide/2
  Divide/1 -> Subtract/1
  Round/1 -> Gain/1
  add/1 -> N/1

== stateflow chart JMAP_Postfilt_SEModelv1d1/JMAP Noise Reduction/Synthesis/Overlap_and_Add/Chart1 ==
  settings: executeAtInitialization=1
  state valid_high
    entry: Pop_Valid=fi(0,0,1,0);
  state Pop_assert
    entry: Pop_Valid=fi(1,0,1,0);
  state valid_low
    entry: Pop_Valid=fi(0,0,1,0);
  state Start_up
    entry: Pop_Valid=fi(0,0,1,0);
  (default) -> Start_up
  Start_up -> valid_low : [valid == 0]
  valid_high -> Pop_assert [order 1] : [valid == 0]
  valid_low -> valid_high [order 1] : [valid == 1]
  valid_low -> valid_low [order 2] : [valid == 0]
  valid_high -> valid_high [order 2] : [valid == 1]
  data: valid input; Pop_Valid output

== matlab function JMAP_Postfilt_SEModelv1d1/JMAP Noise Reduction/Synthesis/Overlap_and_Add/FIFO_Write_Select ==
  data: fifo_counter input; valid_1 output; valid_signal input; valid_2 output; valid_3 output; valid_4 output
function [valid_1, valid_2, valid_3, valid_4] = fcn(fifo_counter, valid_signal)
%#codegen



switch fifo_counter
    case 0
        valid_1 = valid_signal;
        valid_2 = false;
        valid_3 = false;
        valid_4 = false;
    case 1
        valid_1 = false;
        valid_2 = valid_signal;
        valid_3 = false;
        valid_4 = false;
    case 2
        valid_1 = false;
        valid_2 = false;
        valid_3 = valid_signal;
        valid_4 = false;
    case 3
        valid_1 = false;
        valid_2 = false;
        valid_3 = false;
        valid_4 = valid_signal;
    otherwise
        valid_1 = false;
        valid_2 = false;
        valid_3 = false;
        valid_4 = false;
       
end

== stateflow chart JMAP_Postfilt_SEModelv1d1/JMAP Noise Reduction/Synthesis/Overlap_and_Add/Chart2 ==
  settings: executeAtInitialization=1
  state valid_high
    entry: Pop_Valid=fi(0,0,1,0);
  state Pop_assert
    entry: Pop_Valid=fi(1,0,1,0);
  state valid_low
    entry: Pop_Valid=fi(0,0,1,0);
  state Start_up
    entry: Pop_Valid=fi(0,0,1,0);
  (default) -> Start_up
  Start_up -> valid_low : [valid == 0]
  valid_high -> Pop_assert [order 1] : [valid == 0]
  valid_low -> valid_high [order 1] : [valid == 1]
  valid_low -> valid_low [order 2] : [valid == 0]
  valid_high -> valid_high [order 2] : [valid == 1]
  data: valid input; Pop_Valid output

== stateflow chart JMAP_Postfilt_SEModelv1d1/JMAP Noise Reduction/Synthesis/Overlap_and_Add/Chart3 ==
  settings: executeAtInitialization=1
  state valid_high
    entry: Pop_Valid=fi(0,0,1,0);
  state Pop_assert
    entry: Pop_Valid=fi(1,0,1,0);
  state valid_low
    entry: Pop_Valid=fi(0,0,1,0);
  state Start_up
    entry: Pop_Valid=fi(0,0,1,0);
  (default) -> Start_up
  Start_up -> valid_low : [valid == 0]
  valid_high -> Pop_assert [order 1] : [valid == 0]
  valid_low -> valid_high [order 1] : [valid == 1]
  valid_low -> valid_low [order 2] : [valid == 0]
  valid_high -> valid_high [order 2] : [valid == 1]
  data: valid input; Pop_Valid output

== stateflow chart JMAP_Postfilt_SEModelv1d1/JMAP Noise Reduction/Synthesis/Overlap_and_Add/Chart ==
  settings: executeAtInitialization=1
  state valid_high
    entry: Pop_Valid=fi(0,0,1,0);
  state Pop_assert
    entry: Pop_Valid=fi(1,0,1,0);
  state valid_low
    entry: Pop_Valid=fi(0,0,1,0);
  state Start_up
    entry: Pop_Valid=fi(0,0,1,0);
  (default) -> Start_up
  Start_up -> valid_low : [valid == 0]
  valid_high -> Pop_assert [order 1] : [valid == 0]
  valid_low -> valid_high [order 1] : [valid == 1]
  valid_low -> valid_low [order 2] : [valid == 0]
  valid_high -> valid_high [order 2] : [valid == 1]
  data: valid input; Pop_Valid output
